simulink model "encoder_sim"  (Simulink 7.1)
settings: Solver=FixedStepDiscrete  StartTime=0.0  StopTime=60  RelTol=1e-3
libraries: arduino_io_lib x4, simulink x1
settings Model: Creator=gcampa  LastModifiedBy=gcampa
settings OptimizationCC: InitFltsAndDblsToZero=off
settings DebuggingCC: StrictBusMsg=ErrorLevel1
settings GRTTargetCC: CPPClassGenCompliant=off

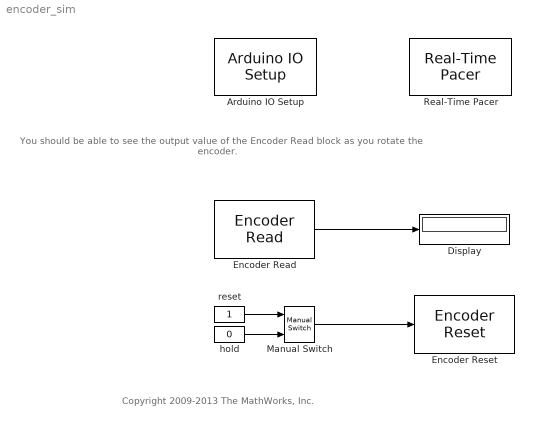
== system encoder_sim ==
  note: You should be able to see the output value of the Encoder Read
      | block as you rotate the encoder.
  note: Copyright 2009-2013 The MathWorks, Inc.
  Arduino IO Setup : arduino_io_lib/Arduino IO Setup  Priority=3  arduinoVar=Temporary arduino variable: Arduino2  workspaceVarName=b  comPort=COM17
  Display : Display
  Encoder Read : arduino_io_lib/Encoder Read  arduinoVar=Temporary arduino variable: Arduino2  encNum=1  pinA=3  pinB=2  DbDl=17  T=0.2
  Encoder Reset : arduino_io_lib/Encoder Reset  arduinoVar=Temporary arduino variable: Arduino2  encNum=1  T=0.2
  Manual Switch : simulink/Signal Routing/Manual Switch  sw=0  action=0  varsize=off
  Real-Time Pacer : arduino_io_lib/Real-Time Pacer  simTimePerRealTime=1
  hold : Constant  Value=0
  reset : Constant
  wires:
  Encoder Read/1 -> Display/1
  reset/1 -> Manual Switch/1
  hold/1 -> Manual Switch/2
  Manual Switch/1 -> Encoder Reset/1
